simulink model "RLC_modelling"  (Simulink 7.2)
settings: Solver=ode45  StartTime=0.0  StopTime=.005  MaxStep=1e-5  RelTol=1e-3
libraries: powerlib x6
settings Model: Creator=ahmed-salah  LastModifiedBy=ahmed-salah

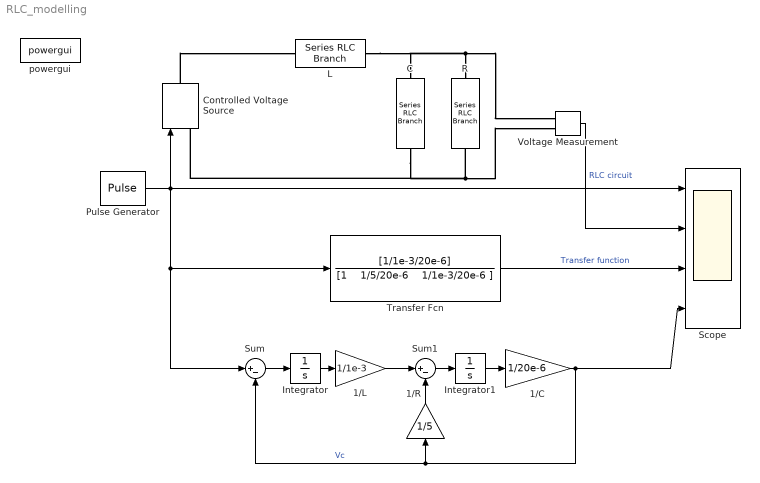
== system RLC_modelling ==
  1/C : Gain  Gain=1/20e-6  ParameterDataType=sfix(16)  ParameterScaling=2^0  OutDataType=sfix(16)  OutScaling=2^0
  1/L : Gain  Gain=1/1e-3  ParameterDataType=sfix(16)  ParameterScaling=2^0  OutDataType=sfix(16)  OutScaling=2^0
  1/R : Gain  Orientation=up  Gain=1/5  ParameterDataType=sfix(16)  ParameterScaling=2^0  OutDataType=sfix(16)  OutScaling=2^0
  C : powerlib/Elements/Series RLC Branch  Orientation=down  DialogController=POWERSYS.PowerSysDialog  PhysicalDomain=powersysdomain  SubClassName=unknown  LeftPortType=p1  RightPortType=p1  LConnTagsString=__new0  RConnTagsString=__new0  BranchType=C  Resistance=1  Inductance=1e-3  SetiL0=off  InitialCurrent=0  Capacitance=20e-6  Setx0=off  InitialVoltage=0  Measurements=None
  Controlled Voltage Source : powerlib/Electrical Sources/Controlled Voltage Source  Orientation=up  DialogController=POWERSYS.PowerSysDialog  SystemSampleTime=-1  Initialize=on  Source_Type=AC  Amplitude=0  Phase=0  Frequency=0  Measurements=None
  Integrator : Integrator
  Integrator1 : Integrator
  L : powerlib/Elements/Series RLC Branch  DialogController=POWERSYS.PowerSysDialog  PhysicalDomain=powersysdomain  SubClassName=unknown  LeftPortType=p1  RightPortType=p1  LConnTagsString=__new0  RConnTagsString=__new0  BranchType=L  Resistance=1  Inductance=1e-3  SetiL0=off  InitialCurrent=0  Capacitance=1e-6  Setx0=off  InitialVoltage=0  Measurements=None
  Pulse Generator : DiscretePulseGenerator  PulseType=Time based  Amplitude=100  Period=1/10e3  PulseWidth=80
  R : powerlib/Elements/Series RLC Branch  Orientation=down  DialogController=POWERSYS.PowerSysDialog  PhysicalDomain=powersysdomain  SubClassName=unknown  LeftPortType=p1  RightPortType=p1  LConnTagsString=__new0  RConnTagsString=__new0  BranchType=R  Resistance=5  Inductance=1e-3  SetiL0=off  InitialCurrent=0  Capacitance=100e-6  Setx0=off  InitialVoltage=0  Measurements=Branch voltage and current
  Scope : Scope  NumInputPorts=4
      settings: TimeRange=0.005  YMin=0~0~0~0  YMax=100~100~100~100
  Sum : Sum  Inputs=|+-  OutDataType=sfix(16)  OutScaling=2^0
  Sum1 : Sum  Inputs=|+-  OutDataType=sfix(16)  OutScaling=2^0
  Transfer Fcn : TransferFcn  Numerator=[1/1e-3/20e-6]  Denominator="[1    1/5/20e-6    1/1e-3/20e-6 ]"
  Voltage Measurement : powerlib/Measurements/Voltage Measurement  DialogController=POWERSYS.PowerSysDialog  SystemSampleTime=-1  PhasorSimulation=off  OutputType=Complex  PSBequivalent=0
  powergui : powerlib/powergui  SystemSampleTime=-1  SimulationMode=Continuous  SampleTime=50e-6  frequency=60  SPID=off  DisableSnubberDevices=off  DisableRonSwitches=off  DisableVfSwitches=off  SwTol=0  Interpol=off  frequencyindice=0  echomessages=off  HookPort=off  FunctionMessages=off  EnableUseOfTLC=off  x0status=blocks  RestoreLinks=warning  Frange=[0:2:500]  Ylog=off  Xlog=on  ShowGrid=off  save=off  variable=ZData  ZoomFFT=on  StartTime=0.0  cycles=1  DisplayStyle=1  fundamental=60  FreqAxis=off  MaxFrequency=1000  frequencyindicesteady=1  RmsSteady=1  display=off  Ts=0  methode=off
  wires:
  Pulse Generator/1 -> Scope/1, Controlled Voltage Source/1, Sum/1, Transfer Fcn/1
  Voltage Measurement/1 -> Scope/2  "RLC circuit"
  Sum/1 -> Integrator/1
  Integrator/1 -> 1/L/1
  1/L/1 -> Sum1/1
  Sum1/1 -> Integrator1/1
  Integrator1/1 -> 1/C/1
  1/C/1 -> Sum/2, 1/R/1, Scope/4  "Vc"
  1/R/1 -> Sum1/2
  Transfer Fcn/1 -> Scope/3  "Transfer function"
  connections:
  Controlled Voltage Source/RConn1 -- L/LConn1
  C/RConn1 -- Controlled Voltage Source/LConn1 -- R/RConn1 -- Voltage Measurement/LConn2
  L/RConn1 -- C/LConn1 -- R/LConn1 -- Voltage Measurement/LConn1
